simulink model "test_pi_av_flocking_xy_gazebo_2023a"  (R2023a)
settings: Solver=FixedStepAuto  StartTime=0.0  StopTime=inf  FixedStep=0.07  RelTol=1e-3
undefined symbols (not defined in the file or in its folder): angular, DiscIntNeverNeededParam, linear
libraries: ros2lib x14, simulink x4, robotcorelib x4
(part 1 of 2)
settings Model: Creator=johvany  LastModifiedBy=l15
settings OptimizationCC: EnhancedBackFolding=on  PassReuseOutputArgsThreshold=0  ZeroExternalMemoryAtStartup=off  ZeroInternalMemoryAtStartup=off  MaxStackSize=64  OptimizeBlockOrder=speed  DifferentSizesBufferReuse=on  OptimizationCustomize=off
settings DebuggingCC: ParameterTunabilityLossMsg=error  UnderSpecifiedDimensionMsg=warning
settings HardwareCC: ProdBitPerLong=64  ProdHWDeviceType=Intel->x86-64 (Linux 64)  UseEmbeddedCoderFeatures=off
settings SFSimCC: MATLABDynamicMemAlloc=off
settings RTWCC: Description=Embedded Coder  SystemTargetFile=ert.tlc  HardwareBoard=Robot Operating System 2 (ROS 2)  TLCOptions="-aInlineSetEventsForThisBaseRateFcn=TLC_FALSE -aSuppressMultiTaskScheduler=TLC_FALSE  -aRateBasedStepFcn=0"  TemplateMakefile=ert_default_tmf  Toolchain=Colcon Tools  TargetLang=C++
settings CodeAppCC: ForceParamTrailComments=on  OperatorAnnotations=on
settings ERTTargetCC: ERTCustomFileBanners=off  CodeInterfacePackaging=C++ class  SupportContinuousTime=on  SupportNonInlinedSFcns=on  RemoveResetFunc=off  ModelStepFunctionPrototypeControlCompliant=off  RootIOFormat=Structure reference

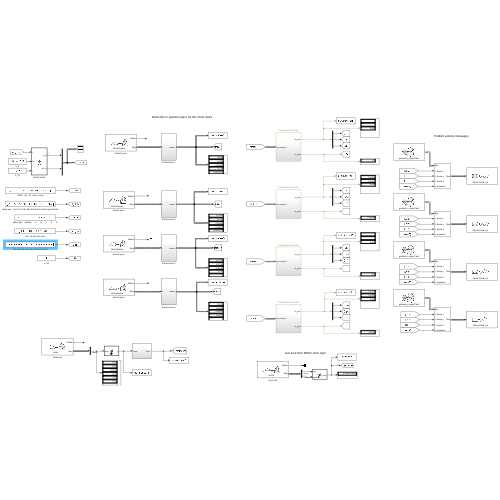
[thumbnail: Simulink's stored preview of the top-level diagram]
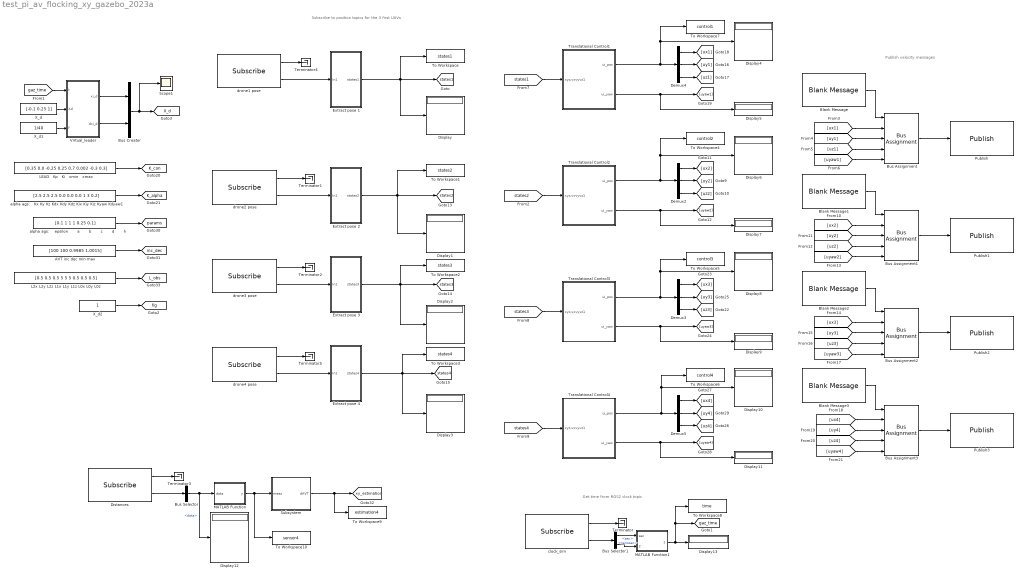
== system test_pi_av_flocking_xy_gazebo_2023a ==
  note: Publish velocity messages
  note: Subscribe to position topics for the 3 first UAVs
  note: Get time from ROS2 clock topic
  AVT inc dec min max : Constant  Value=[100 100 0.9985 1.0015]
  Blank Message{,1..3} (4 alike) : ros2lib/Blank Message  messageClass=Message  entityType=geometry_msgs/Twist  messageType=geometry_msgs/Twist  SampleTime=inf
  Bus Assignment{,1..3} (4 alike) : BusAssignment  AssignedSignals=linear.x,linear.y,linear.z,angular.z
  Bus Creator : BusCreator  Inputs=2
  Bus Selector : BusSelector  OutputSignals=data
  Bus Selector1 : BusSelector  OutputSignals=clock.sec,clock.nanosec
  Demux{2..5} (4 alike) : Demux  Outputs=3
  Display{,1..13} (14 alike) : Display
      Display13 settings: Decimation=4
  Distances : ros2lib/Subscribe  topicSource=Select from ROS network  topic=/dists  messageType=std_msgs/Float32MultiArray  sampleTime=-1  QOSHistory=Keep last  QOSDepth=1  QOSReliability=Reliable  QOSDurability=Volatile
  Extract pose 1 : Subsystem
  Extract pose 2 : Subsystem
  Extract pose 3 : Subsystem
  Extract pose 4 : Subsystem
  L2x L2y L2z L1x L1y L1z L0x L0y L0z : Constant  Value=[0.5 0.5 0.5 5 5 5 0.5 0.5 0.5]
  LEAD   Kp   Ki   xmin   xmax : Constant  Value=[0.35 0.0 -0.25 0.25 0.7 0.002 -0.3 0.3]
  MATLAB Function : MATLAB Function  TreatAsAtomicUnit=on
  MATLAB Function1 : MATLAB Function  TreatAsAtomicUnit=on
  Publish : ros2lib/Publish  topicSource=Select from ROS network  topic=/drone1/cmd_vel  messageType=geometry_msgs/Twist  QOSHistory=Keep last  QOSDepth=1  QOSReliability=Reliable  QOSDurability=Volatile
  Publish1 : ros2lib/Publish  topicSource=Select from ROS network  topic=/drone2/cmd_vel  messageType=geometry_msgs/Twist  QOSHistory=Keep last  QOSDepth=1  QOSReliability=Reliable  QOSDurability=Volatile
  Publish2 : ros2lib/Publish  topicSource=Select from ROS network  topic=/drone3/cmd_vel  messageType=geometry_msgs/Twist  QOSHistory=Keep last  QOSDepth=1  QOSReliability=Reliable  QOSDurability=Volatile
  Publish3 : ros2lib/Publish  topicSource=Select from ROS network  topic=/drone4/cmd_vel  messageType=geometry_msgs/Twist  QOSHistory=Keep last  QOSDepth=1  QOSReliability=Reliable  QOSDurability=Volatile
  Scope1 : Scope
  Subsystem : Subsystem
  Terminator{,1..5} (6 alike) : Terminator
  To Workspace : ToWorkspace  VariableName=states1  SampleTime=-1
  To Workspace1 : ToWorkspace  VariableName=states2  SampleTime=-1
  To Workspace10 : ToWorkspace  VariableName=sensor4  SampleTime=-1
  To Workspace2 : ToWorkspace  VariableName=states3  SampleTime=-1
  To Workspace3 : ToWorkspace  VariableName=states4  SampleTime=-1
  To Workspace4 : ToWorkspace  VariableName=control2  SampleTime=-1
  To Workspace5 : ToWorkspace  VariableName=control3  SampleTime=-1
  To Workspace6 : ToWorkspace  VariableName=control4  SampleTime=-1
  To Workspace7 : ToWorkspace  VariableName=control1  SampleTime=-1
  To Workspace8 : ToWorkspace  VariableName=time  SampleTime=-1
  To Workspace9 : ToWorkspace  VariableName=estimation4  SampleTime=-1
  Translational Control1 : Subsystem
  Translational Control2 : Subsystem
  Translational Control3 : Subsystem
  Translational Control4 : Subsystem
  Virtual_leader : MATLAB Function  TreatAsAtomicUnit=on
  X_d : Constant  Value=[-0.1 0.25 1]
  X_d1 : Constant  Value=1/40
  X_d2 : Constant
  alpha ags:    epsilon       a       b       c       d       h : Constant  Value=[0.1 1 1 1 0.25 0.1]
  alpha ags:   Kx Ky Kz Kdx Kdy Kdz Kix Kiy Kiz Kyaw Kdyaw1 : Constant  Value=[2.5 2.5 2.5 0.0 0.0 0.0 1 3 0.2]
  clock_sim : ros2lib/Subscribe  topicSource=Select from ROS network  topic=/clock  messageType=rosgraph_msgs/Clock  sampleTime=-1  QOSHistory=Keep last  QOSDepth=1  QOSReliability=Reliable  QOSDurability=Volatile
  drone1 pose : ros2lib/Subscribe  topicSource=Select from ROS network  topic=/drone1/pose  messageType=geometry_msgs/PoseStamped  sampleTime=-1  QOSHistory=Keep last  QOSDepth=1  QOSReliability=Reliable  QOSDurability=Volatile
  drone2 pose : ros2lib/Subscribe  topicSource=Select from ROS network  topic=/drone2/pose  messageType=geometry_msgs/PoseStamped  sampleTime=-1  QOSHistory=Keep last  QOSDepth=1  QOSReliability=Reliable  QOSDurability=Volatile
  drone3 pose : ros2lib/Subscribe  topicSource=Select from ROS network  topic=/drone3/pose  messageType=geometry_msgs/PoseStamped  sampleTime=-1  QOSHistory=Keep last  QOSDepth=1  QOSReliability=Reliable  QOSDurability=Volatile
  drone4 pose : ros2lib/Subscribe  topicSource=Select from ROS network  topic=/drone4/pose  messageType=geometry_msgs/PoseStamped  sampleTime=-1  QOSHistory=Keep last  QOSDepth=1  QOSReliability=Reliable  QOSDurability=Volatile
  tag scope: K_alpha=global, K_con=global, L_obs=global, X_d=global, fig=global, gaz_time=global, inc_dec=global, params=global, states1=global, states2=global, states3=global, states4=global, xy_estimation=global
  wires:
  clock_sim/1 -> Terminator/1
  drone2 pose/2 -> Extract pose 2/1(In1)
  drone2 pose/1 -> Terminator1/1
  drone3 pose/2 -> Extract pose 3/1(In1)
  drone3 pose/1 -> Terminator2/1
  Blank Message/1 -> Bus Assignment/1
  Bus Assignment/1 -> Publish/1
  Blank Message1/1 -> Bus Assignment1/1
  Bus Assignment1/1 -> Publish1/1
  Blank Message2/1 -> Bus Assignment2/1
  Bus Assignment2/1 -> Publish2/1
  Blank Message3/1 -> Bus Assignment3/1
  Bus Assignment3/1 -> Publish3/1
  Distances/1 -> Terminator3/1
  Distances/2 -> Bus Selector/1
  Bus Selector/1 -> Display12/1, MATLAB Function/1(data)  "<data>"
  MATLAB Function/1(y) -> To Workspace10/1, Subsystem/1(meas)
  clock_sim/2 -> Bus Selector1/1
  Bus Selector1/1 -> MATLAB Function1/1(sec)  "<sec>"
  Bus Selector1/2 -> MATLAB Function1/2(nanosec)  "<nanosec>"
  Virtual_leader/2(dxi_d) -> Bus Creator/2
  Bus Creator/1 -> Scope1/1, [X_d]
  [gaz_time] -> Virtual_leader/1(t)
  Virtual_leader/1(xi_d) -> Bus Creator/1
  drone1 pose/1 -> Terminator4/1
  drone1 pose/2 -> Extract pose 1/1(In1)
  MATLAB Function1/1(gaz_time) -> To Workspace8/1, [gaz_time], Display13/1
  Extract pose 1/1(states1) -> To Workspace/1, Display/1, [states1]
  [ux1] -> Bus Assignment/2
  [uy1] -> Bus Assignment/3
  [uz1] -> Bus Assignment/4
  [uyaw1] -> Bus Assignment/5
  X_d/1 -> Virtual_leader/2(Xd)
  Extract pose 2/1(states2) -> To Workspace1/1, Display1/1, [states2]
  Extract pose 3/1(states3) -> To Workspace2/1, Display2/1, [states3]
  drone4 pose/2 -> Extract pose 4/1(In1)
  drone4 pose/1 -> Terminator5/1
  Extract pose 4/1(states4) -> To Workspace3/1, Display3/1, [states4]
  [ux2] -> Bus Assignment1/2
  [uy2] -> Bus Assignment1/3
  [uz2] -> Bus Assignment1/4
  [uyaw2] -> Bus Assignment1/5
  [uy3] -> Bus Assignment2/3
  [uyaw3] -> Bus Assignment2/5
  [uz3] -> Bus Assignment2/4
  [ux3] -> Bus Assignment2/2
  [ux4] -> Bus Assignment3/2
  [uy4] -> Bus Assignment3/3
  [uz4] -> Bus Assignment3/4
  [uyaw4] -> Bus Assignment3/5
  Translational Control1/2(ui_yaw) -> Display5/1, [uyaw1]
  Demux4/2 -> [uy1]
  Demux4/3 -> [uz1]
  [states1] -> Translational Control1/1(xyz,vxvyvz1)
  Translational Control1/1(ui_pos) -> Display4/1, To Workspace7/1, Demux4/1
  Demux4/1 -> [ux1]
  LEAD   Kp   Ki   xmin   xmax/1 -> [K_con]
  alpha ags:   Kx Ky Kz Kdx Kdy Kdz Kix Kiy Kiz Kyaw Kdyaw1/1 -> [K_alpha]
  Demux2/1 -> [ux2]
  [states2] -> Translational Control2/1(xyz,vxvyvz1)
  Demux2/3 -> [uz2]
  Demux2/2 -> [uy2]
  Translational Control3/2(ui_yaw) -> Display9/1, [uyaw3]
  Demux3/2 -> [uy3]
  Demux3/3 -> [uz3]
  [states3] -> Translational Control3/1(xyz,vxvyvz1)
  Translational Control3/1(ui_pos) -> To Workspace5/1, Display8/1, Demux3/1
  Demux3/1 -> [ux3]
  Demux5/1 -> [ux4]
  Translational Control4/1(ui_pos) -> To Workspace6/1, Display10/1, Demux5/1
  [states4] -> Translational Control4/1(xyz,vxvyvz1)
  Demux5/3 -> [uz4]
  Demux5/2 -> [uy4]
  Translational Control4/2(ui_yaw) -> Display11/1, [uyaw4]
  alpha ags:    epsilon       a       b       c       d       h/1 -> [params]
  X_d1/1 -> Virtual_leader/3(f)
  AVT inc dec min max/1 -> [inc_dec]
  Subsystem/1(dAVT) -> To Workspace9/1, [xy_estimation]
  L2x L2y L2z L1x L1y L1z L0x L0y L0z/1 -> [L_obs]
  Translational Control2/2(ui_yaw) -> Display7/1, [uyaw2]
  Translational Control2/1(ui_pos) -> To Workspace4/1, Display6/1, Demux2/1
  X_d2/1 -> [fig]

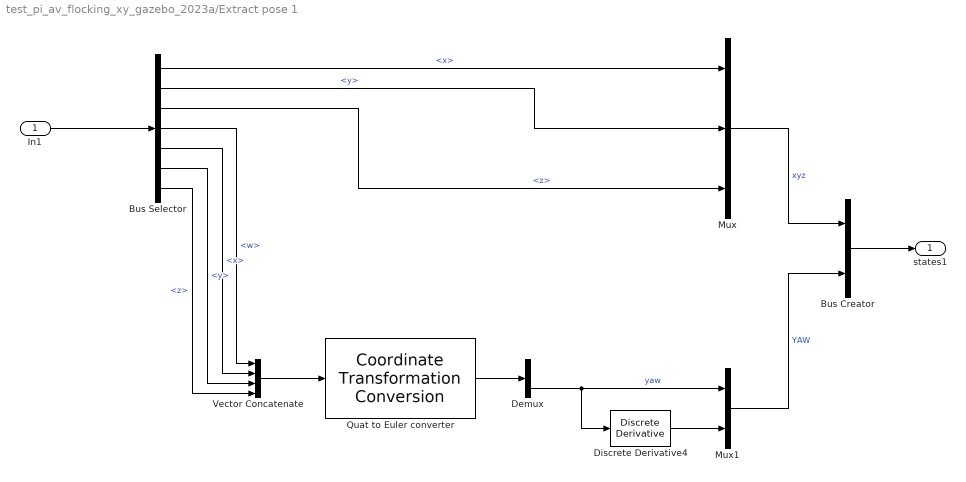
== system test_pi_av_flocking_xy_gazebo_2023a/Extract pose 1 ==
  In1 : Inport
  Bus Creator : BusCreator  Inputs=2
  Bus Selector : BusSelector  OutputSignals=pose.position.x,pose.position.y,pose.position.z,pose.orientation.w,pose.orientation.x,pose.orientation.y,pose.orientation.z
  Demux : Demux  Outputs=3
  Discrete Derivative4 : simulink/Discrete/Discrete Derivative  gainval=1.0  ICPrevScaledInput=0.0  OutMin=[]  OutMax=[]  OutDataType=fixdt(1, 16)  OutScaling=2^-10  DoSatur=off
  Mux : Mux  Inputs=3
  Mux1 : Mux  Inputs=2
  Quat to Euler converter : robotcorelib/Coordinate Transformation Conversion  InputRepresentation=Quaternion  InputEulerSequence=ZYX  ShowTrVecInputPort=on  OutputRepresentation=Euler Angles  OutputEulerSequence=XYZ  ShowTrVecOutputPort=on  SimulateUsing=Interpreted execution
      settings: LibrarySourceBlock=roslib/Utilities/Coordinate Transformation Conversion
  Vector Concatenate : Concatenate  NumInputs=4
  states1 : Outport
  wires:
  Bus Selector/5 -> Vector Concatenate/2  "<x>"
  Quat to Euler converter/1 -> Demux/1
  Bus Selector/6 -> Vector Concatenate/3  "<y>"
  Bus Selector/1 -> Mux/1  "<x>"
  Bus Selector/7 -> Vector Concatenate/4  "<z>"
  Vector Concatenate/1 -> Quat to Euler converter/1
  In1/1 -> Bus Selector/1
  Bus Selector/4 -> Vector Concatenate/1  "<w>"
  Bus Selector/2 -> Mux/2  "<y>"
  Bus Selector/3 -> Mux/3  "<z>"
  Demux/3 -> Discrete Derivative4/1, Mux1/1  "yaw"
  Mux/1 -> Bus Creator/1  "xyz"
  Bus Creator/1 -> states1/1
  Discrete Derivative4/1 -> Mux1/2
  Mux1/1 -> Bus Creator/2  "YAW"

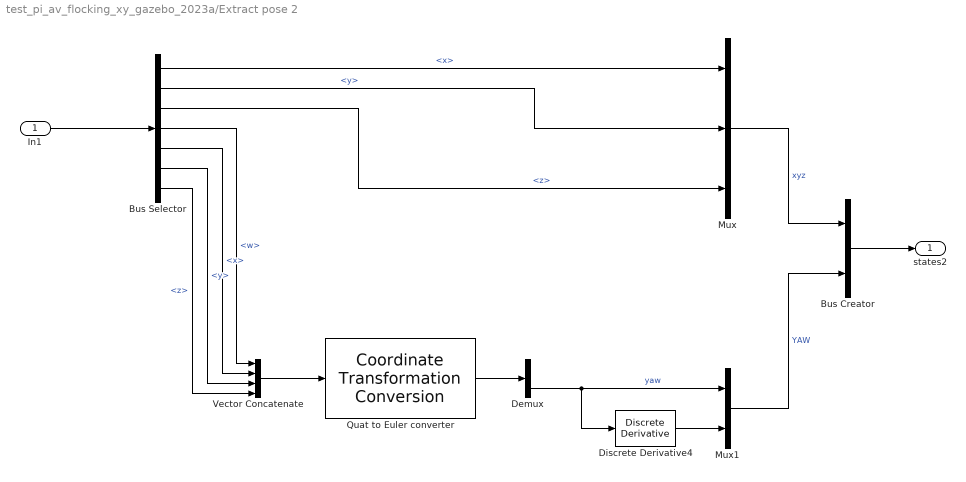
== system test_pi_av_flocking_xy_gazebo_2023a/Extract pose 2 ==
  In1 : Inport
  Bus Creator : BusCreator  Inputs=2
  Bus Selector : BusSelector  OutputSignals=pose.position.x,pose.position.y,pose.position.z,pose.orientation.w,pose.orientation.x,pose.orientation.y,pose.orientation.z
  Demux : Demux  Outputs=3
  Discrete Derivative4 : simulink/Discrete/Discrete Derivative  gainval=1.0  ICPrevScaledInput=0.0  OutMin=[]  OutMax=[]  OutDataType=fixdt(1, 16)  OutScaling=2^-10  DoSatur=off
  Mux : Mux  Inputs=3
  Mux1 : Mux  Inputs=2
  Quat to Euler converter : robotcorelib/Coordinate Transformation Conversion  InputRepresentation=Quaternion  InputEulerSequence=ZYX  ShowTrVecInputPort=on  OutputRepresentation=Euler Angles  OutputEulerSequence=XYZ  ShowTrVecOutputPort=on  SimulateUsing=Interpreted execution
      settings: LibrarySourceBlock=roslib/Utilities/Coordinate Transformation Conversion
  Vector Concatenate : Concatenate  NumInputs=4
  states2 : Outport
  wires:
  Mux1/1 -> Bus Creator/2  "YAW"
  Discrete Derivative4/1 -> Mux1/2
  Bus Creator/1 -> states2/1
  Mux/1 -> Bus Creator/1  "xyz"
  Demux/3 -> Discrete Derivative4/1, Mux1/1  "yaw"
  Bus Selector/3 -> Mux/3  "<z>"
  Bus Selector/2 -> Mux/2  "<y>"
  Bus Selector/4 -> Vector Concatenate/1  "<w>"
  In1/1 -> Bus Selector/1
  Vector Concatenate/1 -> Quat to Euler converter/1
  Bus Selector/7 -> Vector Concatenate/4  "<z>"
  Bus Selector/1 -> Mux/1  "<x>"
  Bus Selector/6 -> Vector Concatenate/3  "<y>"
  Quat to Euler converter/1 -> Demux/1
  Bus Selector/5 -> Vector Concatenate/2  "<x>"

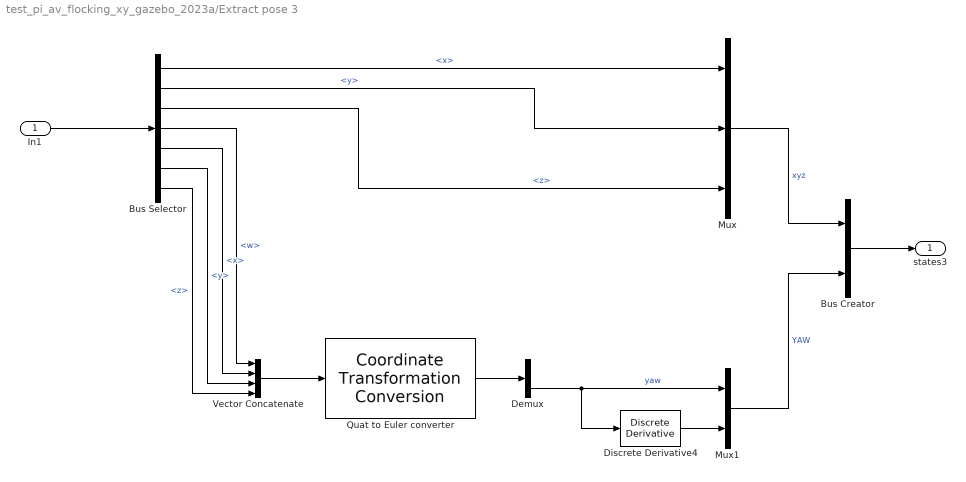
== system test_pi_av_flocking_xy_gazebo_2023a/Extract pose 3 ==
  In1 : Inport
  Bus Creator : BusCreator  Inputs=2
  Bus Selector : BusSelector  OutputSignals=pose.position.x,pose.position.y,pose.position.z,pose.orientation.w,pose.orientation.x,pose.orientation.y,pose.orientation.z
  Demux : Demux  Outputs=3
  Discrete Derivative4 : simulink/Discrete/Discrete Derivative  gainval=1.0  ICPrevScaledInput=0.0  OutMin=[]  OutMax=[]  OutDataType=fixdt(1, 16)  OutScaling=2^-10  DoSatur=off
  Mux : Mux  Inputs=3
  Mux1 : Mux  Inputs=2
  Quat to Euler converter : robotcorelib/Coordinate Transformation Conversion  InputRepresentation=Quaternion  InputEulerSequence=ZYX  ShowTrVecInputPort=on  OutputRepresentation=Euler Angles  OutputEulerSequence=XYZ  ShowTrVecOutputPort=on  SimulateUsing=Interpreted execution
      settings: LibrarySourceBlock=roslib/Utilities/Coordinate Transformation Conversion
  Vector Concatenate : Concatenate  NumInputs=4
  states3 : Outport
  wires:
  Bus Selector/5 -> Vector Concatenate/2  "<x>"
  Quat to Euler converter/1 -> Demux/1
  Bus Selector/6 -> Vector Concatenate/3  "<y>"
  Bus Selector/1 -> Mux/1  "<x>"
  Bus Selector/7 -> Vector Concatenate/4  "<z>"
  Vector Concatenate/1 -> Quat to Euler converter/1
  In1/1 -> Bus Selector/1
  Bus Selector/4 -> Vector Concatenate/1  "<w>"
  Bus Selector/2 -> Mux/2  "<y>"
  Bus Selector/3 -> Mux/3  "<z>"
  Demux/3 -> Discrete Derivative4/1, Mux1/1  "yaw"
  Mux/1 -> Bus Creator/1  "xyz"
  Bus Creator/1 -> states3/1
  Discrete Derivative4/1 -> Mux1/2
  Mux1/1 -> Bus Creator/2  "YAW"

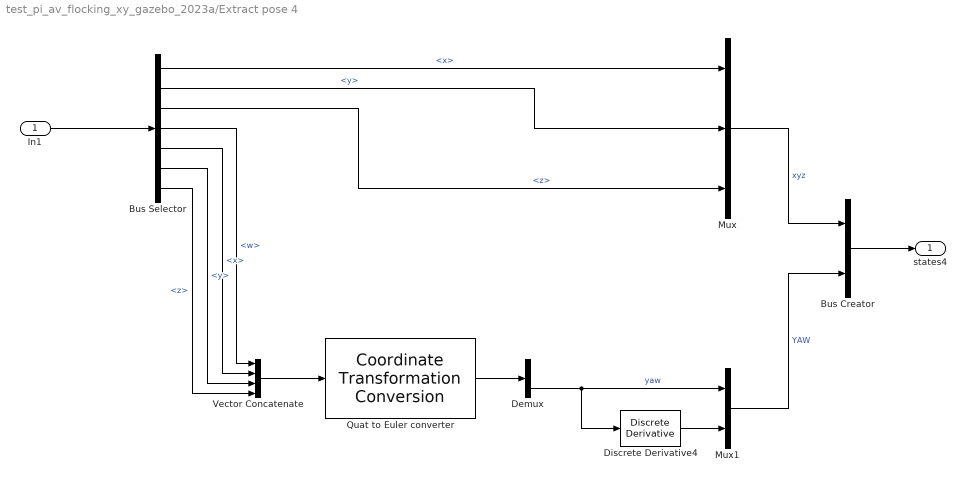
== system test_pi_av_flocking_xy_gazebo_2023a/Extract pose 4 ==
  In1 : Inport
  Bus Creator : BusCreator  Inputs=2
  Bus Selector : BusSelector  OutputSignals=pose.position.x,pose.position.y,pose.position.z,pose.orientation.w,pose.orientation.x,pose.orientation.y,pose.orientation.z
  Demux : Demux  Outputs=3
  Discrete Derivative4 : simulink/Discrete/Discrete Derivative  gainval=1.0  ICPrevScaledInput=0.0  OutMin=[]  OutMax=[]  OutDataType=fixdt(1, 16)  OutScaling=2^-10  DoSatur=off
  Mux : Mux  Inputs=3
  Mux1 : Mux  Inputs=2
  Quat to Euler converter : robotcorelib/Coordinate Transformation Conversion  InputRepresentation=Quaternion  InputEulerSequence=ZYX  ShowTrVecInputPort=on  OutputRepresentation=Euler Angles  OutputEulerSequence=XYZ  ShowTrVecOutputPort=on  SimulateUsing=Interpreted execution
      settings: LibrarySourceBlock=roslib/Utilities/Coordinate Transformation Conversion
  Vector Concatenate : Concatenate  NumInputs=4
  states4 : Outport
  wires:
  Mux1/1 -> Bus Creator/2  "YAW"
  Discrete Derivative4/1 -> Mux1/2
  Bus Creator/1 -> states4/1
  Mux/1 -> Bus Creator/1  "xyz"
  Demux/3 -> Discrete Derivative4/1, Mux1/1  "yaw"
  Bus Selector/3 -> Mux/3  "<z>"
  Bus Selector/2 -> Mux/2  "<y>"
  Bus Selector/4 -> Vector Concatenate/1  "<w>"
  In1/1 -> Bus Selector/1
  Vector Concatenate/1 -> Quat to Euler converter/1
  Bus Selector/7 -> Vector Concatenate/4  "<z>"
  Bus Selector/1 -> Mux/1  "<x>"
  Bus Selector/6 -> Vector Concatenate/3  "<y>"
  Quat to Euler converter/1 -> Demux/1
  Bus Selector/5 -> Vector Concatenate/2  "<x>"

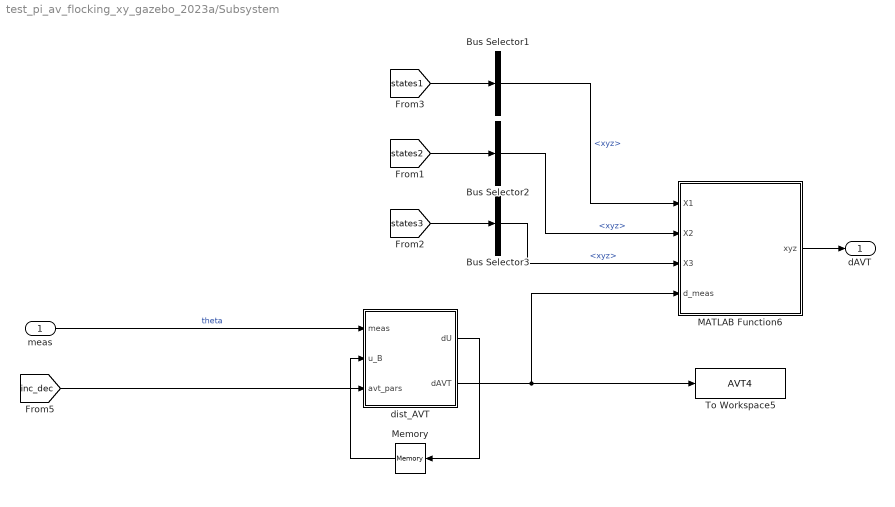
== system test_pi_av_flocking_xy_gazebo_2023a/Subsystem ==
  meas : Inport
  Bus Selector1 : BusSelector  OutputSignals=xyz
  Bus Selector2 : BusSelector  OutputSignals=xyz
  Bus Selector3 : BusSelector  OutputSignals=xyz
  MATLAB Function6 : MATLAB Function  TreatAsAtomicUnit=on
  Memory : Memory  InitialCondition=[1 0.5 0 1 0.5 0 1 0.5 0]
  To Workspace5 : ToWorkspace  VariableName=AVT4  SampleTime=-1
  dist_AVT : MATLAB Function  Tag=Outer control  TreatAsAtomicUnit=on
  dAVT : Outport
  wires:
  Memory/1 -> dist_AVT/2(u_B)
  dist_AVT/2(dAVT) -> To Workspace5/1, MATLAB Function6/4(d_meas)
  dist_AVT/1(dU) -> Memory/1
  meas/1 -> dist_AVT/1(meas)  "theta"
  [inc_dec] -> dist_AVT/3(avt_pars)
  MATLAB Function6/1(xyz) -> dAVT/1
  [states1] -> Bus Selector1/1
  Bus Selector1/1 -> MATLAB Function6/1(X1)  "<xyz>"
  [states2] -> Bus Selector2/1
  [states3] -> Bus Selector3/1
  Bus Selector2/1 -> MATLAB Function6/2(X2)  "<xyz>"
  Bus Selector3/1 -> MATLAB Function6/3(X3)  "<xyz>"

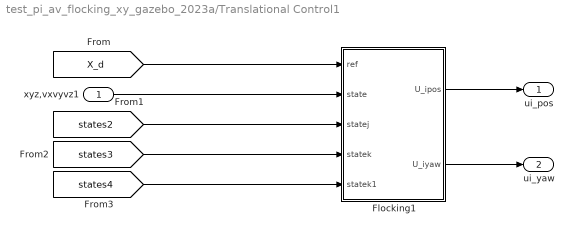
== system test_pi_av_flocking_xy_gazebo_2023a/Translational Control1 ==
  xyz,vxvyvz1 : Inport
  Flocking1 : Subsystem
  ui_pos : Outport  VectorParamsAs1DForOutWhenUnconnected=off
  ui_yaw : Outport  Port=2  VectorParamsAs1DForOutWhenUnconnected=off
  wires:
  [X_d] -> Flocking1/1(ref)
  xyz,vxvyvz1/1 -> Flocking1/2(state)
  [states2] -> Flocking1/3(statej)
  [states3] -> Flocking1/4(statek)
  [states4] -> Flocking1/5(statek1)
  Flocking1/1(U_ipos) -> ui_pos/1
  Flocking1/2(U_iyaw) -> ui_yaw/1

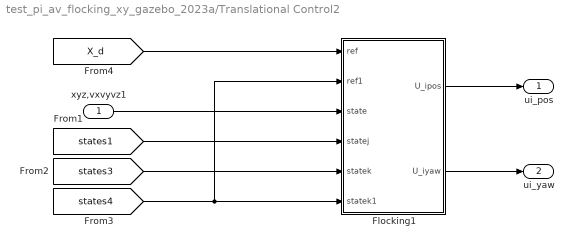
== system test_pi_av_flocking_xy_gazebo_2023a/Translational Control2 ==
  xyz,vxvyvz1 : Inport
  Flocking1 : Subsystem
  ui_pos : Outport  VectorParamsAs1DForOutWhenUnconnected=off
  ui_yaw : Outport  Port=2  VectorParamsAs1DForOutWhenUnconnected=off
  wires:
  Flocking1/2(U_iyaw) -> ui_yaw/1
  Flocking1/1(U_ipos) -> ui_pos/1
  [states4] -> Flocking1/2(ref1), Flocking1/6(statek1)
  [states3] -> Flocking1/5(statek)
  xyz,vxvyvz1/1 -> Flocking1/3(state)
  [states1] -> Flocking1/4(statej)
  [X_d] -> Flocking1/1(ref)

== system test_pi_av_flocking_xy_gazebo_2023a/Translational Control3 ==
  xyz,vxvyvz1 : Inport
  Flocking1 : Subsystem
  ui_pos : Outport  VectorParamsAs1DForOutWhenUnconnected=off
  ui_yaw : Outport  Port=2  VectorParamsAs1DForOutWhenUnconnected=off
  wires:
  [states1] -> Flocking1/4(statej)
  xyz,vxvyvz1/1 -> Flocking1/3(state)
  [states2] -> Flocking1/5(statek)
  [states4] -> Flocking1/2(ref1), Flocking1/6(statek1)
  Flocking1/1(U_ipos) -> ui_pos/1
  Flocking1/2(U_iyaw) -> ui_yaw/1
  [X_d] -> Flocking1/1(ref)

== system test_pi_av_flocking_xy_gazebo_2023a/Translational Control4 ==
  xyz,vxvyvz1 : Inport
  Flocking1 : Subsystem
  ui_pos : Outport  VectorParamsAs1DForOutWhenUnconnected=off
  ui_yaw : Outport  Port=2  VectorParamsAs1DForOutWhenUnconnected=off
  wires:
  Flocking1/2(U_iyaw) -> ui_yaw/1
  Flocking1/1(U_ipos) -> ui_pos/1
  [states3] -> Flocking1/6(statek1)
  [states2] -> Flocking1/5(statek)
  [states1] -> Flocking1/2(ref1), Flocking1/4(statej)
  xyz,vxvyvz1/1 -> Flocking1/3(state)
  [X_d] -> Flocking1/1(ref)

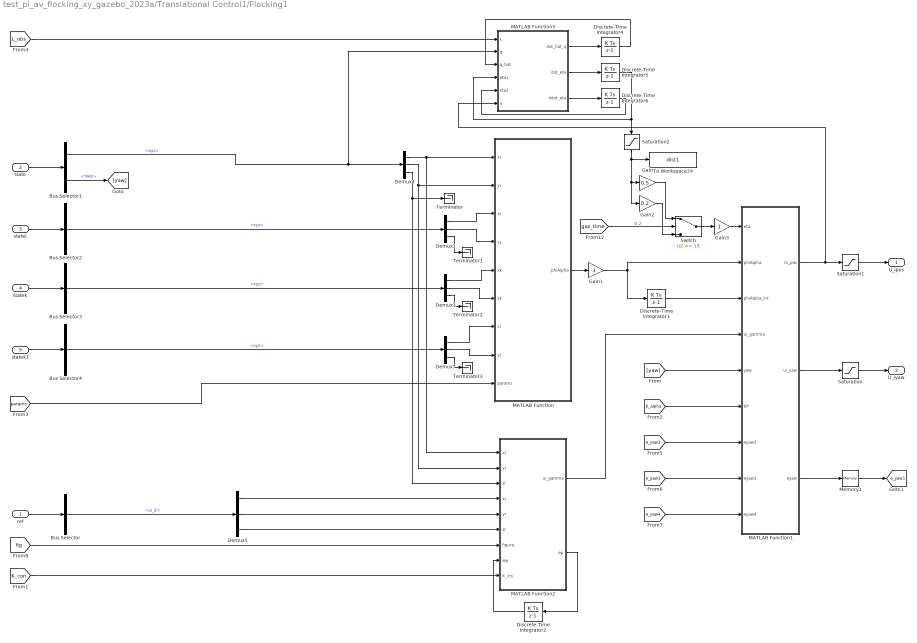
== system test_pi_av_flocking_xy_gazebo_2023a/Translational Control1/Flocking1 ==
  note: 0.2
  ref : Inport
  state : Inport  Port=2
  statej : Inport  Port=3
  statek : Inport  Port=4
  statek1 : Inport  Port=5
  Bus Selector : BusSelector  OutputSignals=xi_d
  Bus Selector1 : BusSelector  OutputSignals=xyz,YAW
  Bus Selector2 : BusSelector  OutputSignals=xyz
  Bus Selector3 : BusSelector  OutputSignals=xyz
  Bus Selector4 : BusSelector  OutputSignals=xyz
  Demux{1,3..5,7} (5 alike) : Demux  Outputs=3
  Discrete-Time Integrator1 : DiscreteIntegrator  SampleTime=-1  LimitOutput=on  UpperSaturationLimit=5  LowerSaturationLimit=-5  ICPrevOutput=DiscIntNeverNeededParam  ICPrevScaledInput=DiscIntNeverNeededParam
  Discrete-Time Integrator2 : DiscreteIntegrator  SampleTime=-1  LimitOutput=on  UpperSaturationLimit=2  LowerSaturationLimit=-2  ICPrevOutput=DiscIntNeverNeededParam  ICPrevScaledInput=DiscIntNeverNeededParam
  Discrete-Time Integrator4 : DiscreteIntegrator  SampleTime=-1  LimitOutput=on  UpperSaturationLimit=0.15  LowerSaturationLimit=-0.15  ICPrevOutput=DiscIntNeverNeededParam  ICPrevScaledInput=DiscIntNeverNeededParam
  Discrete-Time Integrator5 : DiscreteIntegrator  SampleTime=-1  LimitOutput=on  UpperSaturationLimit=0.2  LowerSaturationLimit=-0.2  ICPrevOutput=DiscIntNeverNeededParam  ICPrevScaledInput=DiscIntNeverNeededParam
  Discrete-Time Integrator6 : DiscreteIntegrator  SampleTime=-1  LimitOutput=on  UpperSaturationLimit=0.05  LowerSaturationLimit=-0.05  ICPrevOutput=DiscIntNeverNeededParam  ICPrevScaledInput=DiscIntNeverNeededParam
  Gain : Gain  Gain=0.5
  Gain1 : Gain  Gain=-1
  Gain2 : Gain  Gain=0.2
  Gain3 : Gain
  MATLAB Function : MATLAB Function  TreatAsAtomicUnit=on
  MATLAB Function1 : MATLAB Function  TreatAsAtomicUnit=on
  MATLAB Function2 : MATLAB Function  TreatAsAtomicUnit=on
  MATLAB Function5 : MATLAB Function  TreatAsAtomicUnit=on
  Memory1 : Memory  InitialCondition=1
  Saturation : Saturate  UpperLimit=0.9  LowerLimit=-0.9
  Saturation1 : Saturate  UpperLimit=0.95  LowerLimit=-0.95
  Saturation2 : Saturate  UpperLimit=1  LowerLimit=-1
  Switch : Switch  Threshold=15  SaturateOnIntegerOverflow=off  InputSameDT=off
  Terminator{,1..3} (4 alike) : Terminator
  To Workspace24 : ToWorkspace  VariableName=dist1  SampleTime=-1
  U_ipos : Outport  VectorParamsAs1DForOutWhenUnconnected=off
  U_iyaw : Outport  Port=2  VectorParamsAs1DForOutWhenUnconnected=off
  tag scope: e_yaw1=global
  wires:
  ref/1 -> Bus Selector/1
  state/1 -> Bus Selector1/1
  Bus Selector/1 -> Demux5/1  "<xi_d>"
  statej/1 -> Bus Selector2/1
  Bus Selector2/1 -> Demux1/1  "<xyz>"
  Demux4/1 -> MATLAB Function2/1(xi), MATLAB Function/1(xi)
  Demux4/2 -> MATLAB Function2/2(yi), MATLAB Function/2(yi)
  Demux1/1 -> MATLAB Function/3(xj)
  Demux1/2 -> MATLAB Function/4(yj)
  Discrete-Time Integrator1/1 -> MATLAB Function1/3(phiAlpha_int)
  MATLAB Function2/1(ui_gamma) -> MATLAB Function1/4(ui_gamma)
  statek/1 -> Bus Selector3/1
  Demux3/1 -> MATLAB Function/5(xk)
  Demux3/2 -> MATLAB Function/6(yk)
  Bus Selector3/1 -> Demux3/1  "<xyz>"
  MATLAB Function/1(phiAlpha) -> Gain1/1
  Demux5/1 -> MATLAB Function2/4(xr)
  Demux5/2 -> MATLAB Function2/5(yr)
  Demux4/3 -> Terminator/1, MATLAB Function2/3(zi)
  Demux3/3 -> Terminator2/1
  MATLAB Function1/1(Ui_pos) -> MATLAB Function5/6(u), Saturation1/1
  Demux1/3 -> Terminator1/1
  statek1/1 -> Bus Selector4/1
  Demux7/1 -> MATLAB Function/7(xl)
  Demux7/2 -> MATLAB Function/8(yl)
  Demux7/3 -> Terminator3/1
  Bus Selector4/1 -> Demux7/1  "<xyz>"
  Bus Selector1/1 -> MATLAB Function5/2(q), Demux4/1  "<xyz>"
  Bus Selector1/2 -> [yaw]  "<YAW>"
  [yaw] -> MATLAB Function1/5(yaw)
  MATLAB Function1/2(ui_yaw) -> Saturation/1
  MATLAB Function2/2(ep) -> Discrete-Time Integrator2/1
  Discrete-Time Integrator2/1 -> MATLAB Function2/8(iep)
  [K_con] -> MATLAB Function2/9(K_cts)
  MATLAB Function1/3(eyaw) -> Memory1/1
  [K_alpha] -> MATLAB Function1/6(KP)
  [params] -> MATLAB Function/9(params)
  MATLAB Function5/1(dot_hat_q) -> Discrete-Time Integrator4/1
  Discrete-Time Integrator4/1 -> MATLAB Function5/3(q_hat)
  [L_obs] -> MATLAB Function5/1(L)
  MATLAB Function5/2(dot_eta) -> Discrete-Time Integrator5/1
  MATLAB Function5/3(ddot_eta) -> Discrete-Time Integrator6/1
  Discrete-Time Integrator5/1 -> Saturation2/1, MATLAB Function5/4(eta1)
  Discrete-Time Integrator6/1 -> MATLAB Function5/5(eta2)
  [e_yaw2] -> MATLAB Function1/7(eyaw2)
  [e_yaw3] -> MATLAB Function1/8(eyaw3)
  [e_yaw4] -> MATLAB Function1/9(eyaw4)
  Memory1/1 -> [e_yaw1]
  Saturation/1 -> U_iyaw/1
  Demux5/3 -> MATLAB Function2/6(zr)
  [fig] -> MATLAB Function2/7(figure)
  Gain1/1 -> MATLAB Function1/2(phiAlpha), Discrete-Time Integrator1/1
  Saturation1/1 -> U_ipos/1
  Saturation2/1 -> To Workspace24/1, Gain2/1, Gain/1
  [gaz_time] -> Switch/2
  Gain/1 -> Switch/1
  Gain2/1 -> Switch/3
  Switch/1 -> Gain3/1
  Gain3/1 -> MATLAB Function1/1(eta)

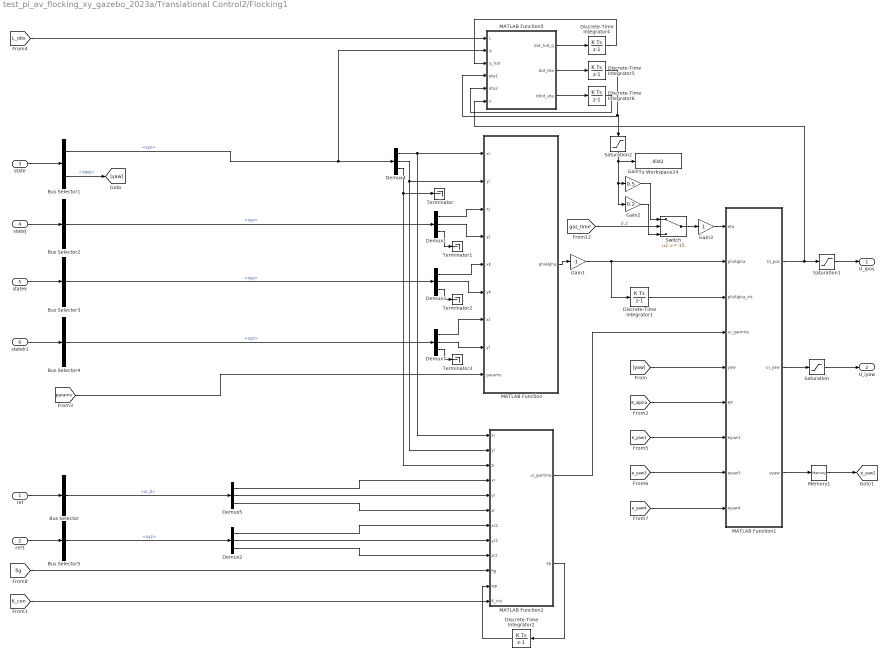
== system test_pi_av_flocking_xy_gazebo_2023a/Translational Control2/Flocking1 ==
  note: 0.2
  ref : Inport
  ref1 : Inport  Port=2
  state : Inport  Port=3
  statej : Inport  Port=4
  statek : Inport  Port=5
  statek1 : Inport  Port=6
  Bus Selector : BusSelector  OutputSignals=xi_d
  Bus Selector1 : BusSelector  OutputSignals=xyz,YAW
  Bus Selector{2..5} (4 alike) : BusSelector  OutputSignals=xyz
  Demux{1..5,7} (6 alike) : Demux  Outputs=3
  Discrete-Time Integrator1 : DiscreteIntegrator  SampleTime=-1  LimitOutput=on  UpperSaturationLimit=5  LowerSaturationLimit=-5  ICPrevOutput=DiscIntNeverNeededParam  ICPrevScaledInput=DiscIntNeverNeededParam
  Discrete-Time Integrator2 : DiscreteIntegrator  SampleTime=-1  LimitOutput=on  UpperSaturationLimit=2  LowerSaturationLimit=-2  ICPrevOutput=DiscIntNeverNeededParam  ICPrevScaledInput=DiscIntNeverNeededParam
  Discrete-Time Integrator4 : DiscreteIntegrator  SampleTime=-1  LimitOutput=on  UpperSaturationLimit=0.15  LowerSaturationLimit=-0.15  ICPrevOutput=DiscIntNeverNeededParam  ICPrevScaledInput=DiscIntNeverNeededParam
  Discrete-Time Integrator5 : DiscreteIntegrator  SampleTime=-1  LimitOutput=on  UpperSaturationLimit=0.2  LowerSaturationLimit=-0.2  ICPrevOutput=DiscIntNeverNeededParam  ICPrevScaledInput=DiscIntNeverNeededParam
  Discrete-Time Integrator6 : DiscreteIntegrator  SampleTime=-1  LimitOutput=on  UpperSaturationLimit=0.05  LowerSaturationLimit=-0.05  ICPrevOutput=DiscIntNeverNeededParam  ICPrevScaledInput=DiscIntNeverNeededParam
  Gain : Gain  Gain=0.5
  Gain1 : Gain  Gain=-1
  Gain2 : Gain  Gain=0.2
  Gain3 : Gain
  MATLAB Function : MATLAB Function  TreatAsAtomicUnit=on
  MATLAB Function1 : MATLAB Function  TreatAsAtomicUnit=on
  MATLAB Function2 : MATLAB Function  TreatAsAtomicUnit=on
  MATLAB Function5 : MATLAB Function  TreatAsAtomicUnit=on
  Memory1 : Memory  InitialCondition=1
  Saturation : Saturate  UpperLimit=0.9  LowerLimit=-0.9
  Saturation1 : Saturate  UpperLimit=0.9  LowerLimit=-0.9
  Saturation2 : Saturate  UpperLimit=1  LowerLimit=-1
  Switch : Switch  Threshold=15  SaturateOnIntegerOverflow=off  InputSameDT=off
  Terminator{,1..3} (4 alike) : Terminator
  To Workspace24 : ToWorkspace  VariableName=dist2  SampleTime=-1
  U_ipos : Outport  VectorParamsAs1DForOutWhenUnconnected=off
  U_iyaw : Outport  Port=2  VectorParamsAs1DForOutWhenUnconnected=off
  tag scope: e_yaw2=global
  wires:
  ref/1 -> Bus Selector/1
  state/1 -> Bus Selector1/1
  Bus Selector/1 -> Demux5/1  "<xi_d>"
  statej/1 -> Bus Selector2/1
  Bus Selector2/1 -> Demux1/1  "<xyz>"
  Demux4/1 -> MATLAB Function2/1(xi), MATLAB Function/1(xi)
  Demux4/2 -> MATLAB Function2/2(yi), MATLAB Function/2(yi)
  Demux1/1 -> MATLAB Function/3(xj)
  Demux1/2 -> MATLAB Function/4(yj)
  Discrete-Time Integrator1/1 -> MATLAB Function1/3(phiAlpha_int)
  MATLAB Function2/1(ui_gamma) -> MATLAB Function1/4(ui_gamma)
  statek/1 -> Bus Selector3/1
  Demux3/1 -> MATLAB Function/5(xk)
  Demux3/2 -> MATLAB Function/6(yk)
  Bus Selector3/1 -> Demux3/1  "<xyz>"
  MATLAB Function/1(phiAlpha) -> Gain1/1
  Demux5/1 -> MATLAB Function2/4(xr)
  Demux5/2 -> MATLAB Function2/5(yr)
  Demux4/3 -> Terminator/1, MATLAB Function2/3(zi)
  Demux3/3 -> Terminator2/1
  MATLAB Function1/1(Ui_pos) -> MATLAB Function5/6(u), Saturation1/1
  Demux1/3 -> Terminator1/1
  statek1/1 -> Bus Selector4/1
  Demux7/1 -> MATLAB Function/7(xl)
  Demux7/2 -> MATLAB Function/8(yl)
  Demux7/3 -> Terminator3/1
  Bus Selector4/1 -> Demux7/1  "<xyz>"
  Bus Selector1/2 -> [yaw]  "<YAW>"
  [yaw] -> MATLAB Function1/5(yaw)
  MATLAB Function1/2(ui_yaw) -> Saturation/1
  MATLAB Function2/2(ep) -> Discrete-Time Integrator2/1
  Discrete-Time Integrator2/1 -> MATLAB Function2/11(iep)
  [K_con] -> MATLAB Function2/12(K_cts)
  MATLAB Function1/3(eyaw) -> Memory1/1
  [K_alpha] -> MATLAB Function1/6(KP)
  [params] -> MATLAB Function/9(params)
  [L_obs] -> MATLAB Function5/1(L)
  MATLAB Function5/1(dot_hat_q) -> Discrete-Time Integrator4/1
  Discrete-Time Integrator4/1 -> MATLAB Function5/3(q_hat)
  MATLAB Function5/2(dot_eta) -> Discrete-Time Integrator5/1
  MATLAB Function5/3(ddot_eta) -> Discrete-Time Integrator6/1
  Discrete-Time Integrator6/1 -> MATLAB Function5/5(eta2)
  Bus Selector1/1 -> MATLAB Function5/2(q), Demux4/1  "<xyz>"
  Discrete-Time Integrator5/1 -> Saturation2/1, MATLAB Function5/4(eta1)
  [e_yaw1] -> MATLAB Function1/7(eyaw1)
  [e_yaw3] -> MATLAB Function1/8(eyaw3)
  [e_yaw4] -> MATLAB Function1/9(eyaw4)
  Memory1/1 -> [e_yaw2]
  Saturation/1 -> U_iyaw/1
  Demux5/3 -> MATLAB Function2/6(zr)
  Bus Selector5/1 -> Demux2/1  "<xyz>"
  ref1/1 -> Bus Selector5/1
  Demux2/1 -> MATLAB Function2/7(xr2)
  Demux2/2 -> MATLAB Function2/8(yr2)
  Demux2/3 -> MATLAB Function2/9(zr2)
  [fig] -> MATLAB Function2/10(fig)
  Gain1/1 -> MATLAB Function1/2(phiAlpha), Discrete-Time Integrator1/1
  Saturation1/1 -> U_ipos/1
  Saturation2/1 -> To Workspace24/1, Gain2/1, Gain/1
  Gain2/1 -> Switch/3
  [gaz_time] -> Switch/2
  Gain/1 -> Switch/1
  Switch/1 -> Gain3/1
  Gain3/1 -> MATLAB Function1/1(eta)

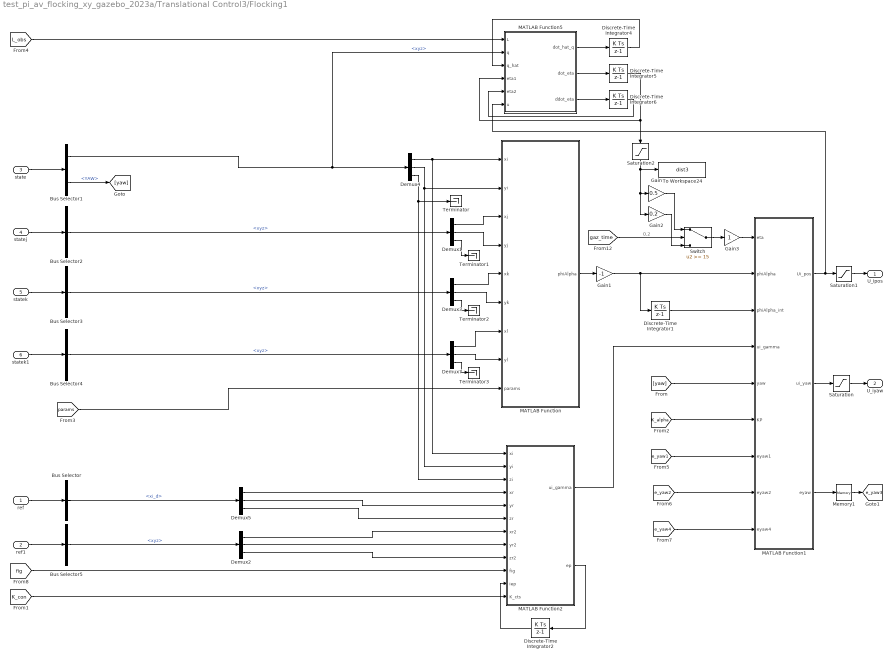
== system test_pi_av_flocking_xy_gazebo_2023a/Translational Control3/Flocking1 ==
  note: 0.2
  ref : Inport
  ref1 : Inport  Port=2
  state : Inport  Port=3
  statej : Inport  Port=4
  statek : Inport  Port=5
  statek1 : Inport  Port=6
  Bus Selector : BusSelector  OutputSignals=xi_d
  Bus Selector1 : BusSelector  OutputSignals=xyz,YAW
  Bus Selector{2..5} (4 alike) : BusSelector  OutputSignals=xyz
  Demux{1..5,7} (6 alike) : Demux  Outputs=3
  Discrete-Time Integrator1 : DiscreteIntegrator  SampleTime=-1  LimitOutput=on  UpperSaturationLimit=5  LowerSaturationLimit=-5  ICPrevOutput=DiscIntNeverNeededParam  ICPrevScaledInput=DiscIntNeverNeededParam
  Discrete-Time Integrator2 : DiscreteIntegrator  SampleTime=-1  LimitOutput=on  UpperSaturationLimit=2  LowerSaturationLimit=-2  ICPrevOutput=DiscIntNeverNeededParam  ICPrevScaledInput=DiscIntNeverNeededParam
  Discrete-Time Integrator4 : DiscreteIntegrator  SampleTime=-1  LimitOutput=on  UpperSaturationLimit=0.15  LowerSaturationLimit=-0.15  ICPrevOutput=DiscIntNeverNeededParam  ICPrevScaledInput=DiscIntNeverNeededParam
  Discrete-Time Integrator5 : DiscreteIntegrator  SampleTime=-1  LimitOutput=on  UpperSaturationLimit=0.2  LowerSaturationLimit=-0.2  ICPrevOutput=DiscIntNeverNeededParam  ICPrevScaledInput=DiscIntNeverNeededParam
  Discrete-Time Integrator6 : DiscreteIntegrator  SampleTime=-1  LimitOutput=on  UpperSaturationLimit=0.05  LowerSaturationLimit=-0.05  ICPrevOutput=DiscIntNeverNeededParam  ICPrevScaledInput=DiscIntNeverNeededParam
  Gain : Gain  Gain=0.5
  Gain1 : Gain  Gain=-1
  Gain2 : Gain  Gain=0.2
  Gain3 : Gain
  MATLAB Function : MATLAB Function  TreatAsAtomicUnit=on
  MATLAB Function1 : MATLAB Function  TreatAsAtomicUnit=on
  MATLAB Function2 : MATLAB Function  TreatAsAtomicUnit=on
  MATLAB Function5 : MATLAB Function  TreatAsAtomicUnit=on
  Memory1 : Memory  InitialCondition=1
  Saturation : Saturate  UpperLimit=0.9  LowerLimit=-0.9
  Saturation1 : Saturate  UpperLimit=0.9  LowerLimit=-0.9
  Saturation2 : Saturate  UpperLimit=1  LowerLimit=-1
  Switch : Switch  Threshold=15  SaturateOnIntegerOverflow=off  InputSameDT=off
  Terminator{,1..3} (4 alike) : Terminator
  To Workspace24 : ToWorkspace  VariableName=dist3  SampleTime=-1
  U_ipos : Outport  VectorParamsAs1DForOutWhenUnconnected=off
  U_iyaw : Outport  Port=2  VectorParamsAs1DForOutWhenUnconnected=off
  tag scope: e_yaw3=global
  wires:
  ref/1 -> Bus Selector/1
  state/1 -> Bus Selector1/1
  Bus Selector/1 -> Demux5/1  "<xi_d>"
  statej/1 -> Bus Selector2/1
  Bus Selector2/1 -> Demux1/1  "<xyz>"
  Demux4/1 -> MATLAB Function2/1(xi), MATLAB Function/1(xi)
  Demux4/2 -> MATLAB Function2/2(yi), MATLAB Function/2(yi)
  Demux1/1 -> MATLAB Function/3(xj)
  Demux1/2 -> MATLAB Function/4(yj)
  Discrete-Time Integrator1/1 -> MATLAB Function1/3(phiAlpha_int)
  MATLAB Function2/1(ui_gamma) -> MATLAB Function1/4(ui_gamma)
  statek/1 -> Bus Selector3/1
  Demux3/1 -> MATLAB Function/5(xk)
  Demux3/2 -> MATLAB Function/6(yk)
  Bus Selector3/1 -> Demux3/1  "<xyz>"
  MATLAB Function/1(phiAlpha) -> Gain1/1
  Demux5/1 -> MATLAB Function2/4(xr)
  Demux5/2 -> MATLAB Function2/5(yr)
  Demux4/3 -> Terminator/1, MATLAB Function2/3(zi)
  Demux3/3 -> Terminator2/1
  MATLAB Function1/1(Ui_pos) -> MATLAB Function5/6(u), Saturation1/1
  Demux1/3 -> Terminator1/1
  statek1/1 -> Bus Selector4/1
  Demux7/1 -> MATLAB Function/7(xl)
  Demux7/2 -> MATLAB Function/8(yl)
  Demux7/3 -> Terminator3/1
  Bus Selector4/1 -> Demux7/1  "<xyz>"
  Bus Selector1/1 -> MATLAB Function5/2(q), Demux4/1  "<xyz>"
  Bus Selector1/2 -> [yaw]  "<YAW>"
  [yaw] -> MATLAB Function1/5(yaw)
  MATLAB Function1/2(ui_yaw) -> Saturation/1
  MATLAB Function2/2(ep) -> Discrete-Time Integrator2/1
  Discrete-Time Integrator2/1 -> MATLAB Function2/11(iep)
  [K_con] -> MATLAB Function2/12(K_cts)
  MATLAB Function1/3(eyaw) -> Memory1/1
  [K_alpha] -> MATLAB Function1/6(KP)
  [params] -> MATLAB Function/9(params)
  Discrete-Time Integrator6/1 -> MATLAB Function5/5(eta2)
  MATLAB Function5/3(ddot_eta) -> Discrete-Time Integrator6/1
  Discrete-Time Integrator4/1 -> MATLAB Function5/3(q_hat)
  MATLAB Function5/2(dot_eta) -> Discrete-Time Integrator5/1
  MATLAB Function5/1(dot_hat_q) -> Discrete-Time Integrator4/1
  [L_obs] -> MATLAB Function5/1(L)
  Discrete-Time Integrator5/1 -> Saturation2/1, MATLAB Function5/4(eta1)
  [e_yaw2] -> MATLAB Function1/8(eyaw2)
  [e_yaw4] -> MATLAB Function1/9(eyaw4)
  [e_yaw1] -> MATLAB Function1/7(eyaw1)
  Memory1/1 -> [e_yaw3]
  Saturation/1 -> U_iyaw/1
  Demux5/3 -> MATLAB Function2/6(zr)
  Bus Selector5/1 -> Demux2/1  "<xyz>"
  ref1/1 -> Bus Selector5/1
  Demux2/3 -> MATLAB Function2/9(zr2)
  Demux2/2 -> MATLAB Function2/8(yr2)
  Demux2/1 -> MATLAB Function2/7(xr2)
  [fig] -> MATLAB Function2/10(fig)
  Gain1/1 -> MATLAB Function1/2(phiAlpha), Discrete-Time Integrator1/1
  Saturation1/1 -> U_ipos/1
  Saturation2/1 -> To Workspace24/1, Gain2/1, Gain/1
  Gain2/1 -> Switch/3
  [gaz_time] -> Switch/2
  Gain/1 -> Switch/1
  Switch/1 -> Gain3/1
  Gain3/1 -> MATLAB Function1/1(eta)

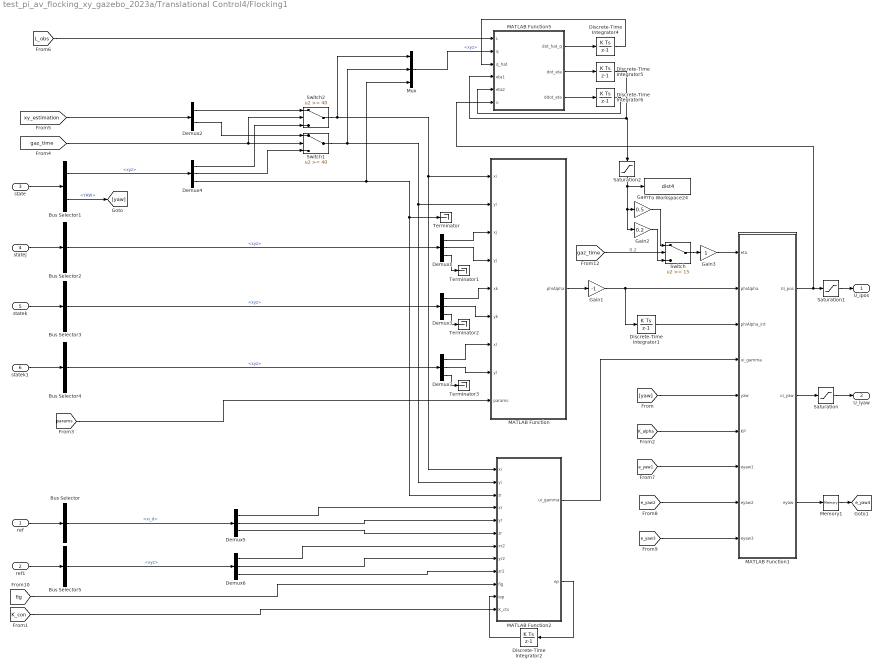
== system test_pi_av_flocking_xy_gazebo_2023a/Translational Control4/Flocking1 ==
  note: 0.2
  ref : Inport
  ref1 : Inport  Port=2
  state : Inport  Port=3
  statej : Inport  Port=4
  statek : Inport  Port=5
  statek1 : Inport  Port=6
  Bus Selector : BusSelector  OutputSignals=xi_d
  Bus Selector1 : BusSelector  OutputSignals=xyz,YAW
  Bus Selector{2..5} (4 alike) : BusSelector  OutputSignals=xyz
  Demux{1,3..7} (6 alike) : Demux  Outputs=3
  Demux2 : Demux  Outputs=2
  Discrete-Time Integrator1 : DiscreteIntegrator  SampleTime=-1  LimitOutput=on  UpperSaturationLimit=5  LowerSaturationLimit=-5  ICPrevOutput=DiscIntNeverNeededParam  ICPrevScaledInput=DiscIntNeverNeededParam
  Discrete-Time Integrator2 : DiscreteIntegrator  SampleTime=-1  LimitOutput=on  UpperSaturationLimit=2  LowerSaturationLimit=-2  ICPrevOutput=DiscIntNeverNeededParam  ICPrevScaledInput=DiscIntNeverNeededParam
  Discrete-Time Integrator4 : DiscreteIntegrator  SampleTime=-1  LimitOutput=on  UpperSaturationLimit=0.15  LowerSaturationLimit=-0.15  ICPrevOutput=DiscIntNeverNeededParam  ICPrevScaledInput=DiscIntNeverNeededParam
  Discrete-Time Integrator5 : DiscreteIntegrator  SampleTime=-1  LimitOutput=on  UpperSaturationLimit=0.2  LowerSaturationLimit=-0.2  ICPrevOutput=DiscIntNeverNeededParam  ICPrevScaledInput=DiscIntNeverNeededParam
  Discrete-Time Integrator6 : DiscreteIntegrator  SampleTime=-1  LimitOutput=on  UpperSaturationLimit=0.05  LowerSaturationLimit=-0.05  ICPrevOutput=DiscIntNeverNeededParam  ICPrevScaledInput=DiscIntNeverNeededParam
  Gain : Gain  Gain=0.5
  Gain1 : Gain  Gain=-1
  Gain2 : Gain  Gain=0.2
  Gain3 : Gain
  MATLAB Function : MATLAB Function  TreatAsAtomicUnit=on
  MATLAB Function1 : MATLAB Function  TreatAsAtomicUnit=on
  MATLAB Function2 : MATLAB Function  TreatAsAtomicUnit=on
  MATLAB Function5 : MATLAB Function  TreatAsAtomicUnit=on
  Memory1 : Memory  InitialCondition=1
  Mux : Mux  Inputs=3
  Saturation : Saturate  UpperLimit=0.9  LowerLimit=-0.9
  Saturation1 : Saturate  UpperLimit=0.9  LowerLimit=-0.9
  Saturation2 : Saturate  UpperLimit=1  LowerLimit=-1
  Switch : Switch  Threshold=15  SaturateOnIntegerOverflow=off  InputSameDT=off
  Switch1 : Switch  Threshold=40  SaturateOnIntegerOverflow=off  InputSameDT=off
  Switch2 : Switch  Threshold=40  SaturateOnIntegerOverflow=off  InputSameDT=off
  Terminator{,1..3} (4 alike) : Terminator
  To Workspace24 : ToWorkspace  VariableName=dist4  SampleTime=-1
  U_ipos : Outport  VectorParamsAs1DForOutWhenUnconnected=off
  U_iyaw : Outport  Port=2  VectorParamsAs1DForOutWhenUnconnected=off
  tag scope: e_yaw4=global
  wires:
  ref/1 -> Bus Selector/1
  state/1 -> Bus Selector1/1
  Bus Selector/1 -> Demux5/1  "<xi_d>"
  statej/1 -> Bus Selector2/1
  Bus Selector2/1 -> Demux1/1  "<xyz>"
  Demux1/1 -> MATLAB Function/3(xj)
  Demux1/2 -> MATLAB Function/4(yj)
  Discrete-Time Integrator1/1 -> MATLAB Function1/3(phiAlpha_int)
  MATLAB Function2/1(ui_gamma) -> MATLAB Function1/4(ui_gamma)
  statek/1 -> Bus Selector3/1
  Demux3/1 -> MATLAB Function/5(xk)
  Demux3/2 -> MATLAB Function/6(yk)
  Bus Selector3/1 -> Demux3/1  "<xyz>"
  MATLAB Function/1(phiAlpha) -> Gain1/1
  Demux5/1 -> MATLAB Function2/4(xr)
  Demux5/2 -> MATLAB Function2/5(yr)
  Demux4/3 -> Mux/3, Terminator/1, MATLAB Function2/3(zi)
  Demux3/3 -> Terminator2/1
  MATLAB Function1/1(Ui_pos) -> MATLAB Function5/6(u), Saturation1/1
  Demux1/3 -> Terminator1/1
  statek1/1 -> Bus Selector4/1
  Demux7/1 -> MATLAB Function/7(xl)
  Demux7/2 -> MATLAB Function/8(yl)
  Demux7/3 -> Terminator3/1
  Bus Selector4/1 -> Demux7/1  "<xyz>"
  Bus Selector1/2 -> [yaw]  "<YAW>"
  [yaw] -> MATLAB Function1/5(yaw)
  MATLAB Function1/2(ui_yaw) -> Saturation/1
  MATLAB Function2/2(ep) -> Discrete-Time Integrator2/1
  Discrete-Time Integrator2/1 -> MATLAB Function2/11(iep)
  [K_con] -> MATLAB Function2/12(K_cts)
  MATLAB Function1/3(eyaw) -> Memory1/1
  [K_alpha] -> MATLAB Function1/6(KP)
  [params] -> MATLAB Function/9(params)
  Bus Selector1/1 -> Demux4/1  "<xyz>"
  [xy_estimation] -> Demux2/1
  [gaz_time] -> Switch1/2, Switch2/2
  Switch2/1 -> MATLAB Function2/1(xi), MATLAB Function/1(xi), Mux/1
  Switch1/1 -> MATLAB Function/2(yi), MATLAB Function2/2(yi), Mux/2
  Demux2/1 -> Switch2/1
  Demux2/2 -> Switch1/1
  [L_obs] -> MATLAB Function5/1(L)
  Discrete-Time Integrator4/1 -> MATLAB Function5/3(q_hat)
  MATLAB Function5/2(dot_eta) -> Discrete-Time Integrator5/1
  Discrete-Time Integrator5/1 -> Saturation2/1, MATLAB Function5/4(eta1)
  MATLAB Function5/3(ddot_eta) -> Discrete-Time Integrator6/1
  Discrete-Time Integrator6/1 -> MATLAB Function5/5(eta2)
  MATLAB Function5/1(dot_hat_q) -> Discrete-Time Integrator4/1
  Mux/1 -> MATLAB Function5/2(q)  "<xyz>"
  [e_yaw1] -> MATLAB Function1/7(eyaw1)
  [e_yaw2] -> MATLAB Function1/8(eyaw2)
  [e_yaw3] -> MATLAB Function1/9(eyaw3)
  Memory1/1 -> [e_yaw4]
  Demux4/1 -> Switch2/3
  Demux4/2 -> Switch1/3
  Saturation/1 -> U_iyaw/1
  Demux5/3 -> MATLAB Function2/6(zr)
  Bus Selector5/1 -> Demux6/1  "<xyz>"
  ref1/1 -> Bus Selector5/1
  Demux6/2 -> MATLAB Function2/8(yr2)
  Demux6/1 -> MATLAB Function2/7(xr2)
  Demux6/3 -> MATLAB Function2/9(zr2)
  Gain1/1 -> MATLAB Function1/2(phiAlpha), Discrete-Time Integrator1/1
  Saturation1/1 -> U_ipos/1
  [fig] -> MATLAB Function2/10(fig)
  Saturation2/1 -> To Workspace24/1, Gain2/1, Gain/1
  Gain2/1 -> Switch/3
  [gaz_time] -> Switch/2
  Gain/1 -> Switch/1
  Switch/1 -> Gain3/1
  Gain3/1 -> MATLAB Function1/1(eta)

== matlab function test_pi_av_flocking_xy_gazebo_2023a/MATLAB Function ==
  data: data input; y output
function y = fcn(data)

%DATA = data(1:20);
d1 = double(data(4));
d2 = double(data(5));
d3 = double(data(6));
y = [d1;d2;d3];

== matlab function test_pi_av_flocking_xy_gazebo_2023a/Virtual_leader ==
  data: t input; xi_d output; dxi_d output; Xd input; f input
function [xi_d, dxi_d]  = fcn(t, Xd, f)
%#codegen



%f=1/60;    %freq in Hz
radius=1;   %radius in meters

sel=2;      %inputs or parameters dont work! only local vars ...

if sel == 1
    if t < 90
       xd     =  0.4;
       xdotd  =  0;
           
       yd     = 0.4;
       ydotd  = 0;
           
       zd     = 0.7;  
       zdotd  = 0; 
           
       xi_d =[xd; yd; zd];
       dxi_d=[xdotd; ydotd; zdotd]; 
       
    elseif t < 120
        xd     =  0.4;
        xdotd  =  0;
            
        yd     = -0.4;
        ydotd  = 0;
            
        zd     = 0.7;  
        zdotd  = 0; 
            
        xi_d =[xd; yd; zd];
        dxi_d=[xdotd; ydotd; zdotd]; 
        
    else
       xd     = radius*sin(2*pi*f*t);
       xdotd  = radius*2*pi*f*cos(2*pi*f*t);
            
       yd     = radius*cos(2*pi*f*t);
       ydotd  = -radius*2*pi*f*sin(2*pi*f*t);
            
       zd     = 0.7;  %radius*cos(2*pi*f*t) + 5;
       zdotd  = 0;  %-radius*2*pi*f*sin(2*pi*f*t);
           
       xi_d =[xd; yd; zd];
       dxi_d=[xdotd; ydotd; zdotd];
       
    end
end

 if(sel==2)
     xd     =  Xd(1);
     xdotd  =  0;
          
     yd     = Xd(2);
     ydotd  = 0;
          
     zd     = Xd(3);  
     zdotd  = 0; 
          
     xi_d =[xd; yd; zd];
     dxi_d=[xdotd; ydotd; zdotd]; 
     
 end

== matlab function test_pi_av_flocking_xy_gazebo_2023a/Translational Control2/Flocking1/MATLAB Function ==
  data: xi input; yi input; phiAlpha output; xj input; yj input; xk input; yk input; xl input; yl input; params input

function phiAlpha  = phiAlphaFcn(xi, yi, xj, yj, xk, yk, xl, yl, params)
    
    % Flocking parameters
    epsilon = params(1); a = params(2); b = params(3); c = params(4); d = params(5); h = params(6);

    e = abs(a - b) / sqrt(4*a*b) ;

    cAlpha = sigmaNormFun(c, epsilon) ;
    dAlpha = sigmaNormFun(d, epsilon) ;

    %%
    Pi = [xi;yi] ;
    Pj = [xj;yj] ;
    Pk = [xk;yk] ;
    Pl = [xl;yl] ;

    %%
    sigmaNormj = sigmaNormFun(Pj - Pi, epsilon) ;
    nij = gradSigmaFun(Pj - Pi, epsilon) ;
    
    sigmaNormk = sigmaNormFun(Pk - Pi, epsilon) ;
    nik = gradSigmaFun(Pk - Pi, epsilon) ;

    sigmaNorml = sigmaNormFun(Pl - Pi, epsilon) ;
    nil = gradSigmaFun(Pl - Pi, epsilon) ;

    %%
    sigma1j = sigma1Fun(sigmaNormj - dAlpha + e) ;
    sigma1k = sigma1Fun(sigmaNormk - dAlpha + e) ;
    sigma1l = sigma1Fun(sigmaNorml - dAlpha + e) ;
            
    %% Position
    phiAlphaj = 0.5 * bumpFcn(sigmaNormj/cAlpha,h) * ((a+b)*sigma1j + (a-b)) ;
    phiAlphanij = phiAlphaj.* nij ;
    
    phiAlphak = 0.5 * bumpFcn(sigmaNormk/cAlpha,h) * ((a+b)*sigma1k + (a-b)) ;
    phiAlphanik = phiAlphak.* nik ;

    phiAlphal = 0.5 * bumpFcn(sigmaNorml/cAlpha,h) * ((a+b)*sigma1l + (a-b)) ;
    phiAlphanil = phiAlphal.* nil ;

    phiAlpha = phiAlphanij + phiAlphanik + phiAlphanil;

    
end

== matlab function test_pi_av_flocking_xy_gazebo_2023a/Translational Control2/Flocking1/MATLAB Function1 ==
  data: eta input; phiAlpha input; phiAlpha_int input; ui_gamma input; yaw input; Ui_pos output size=3; ui_yaw output; KP input; eyaw output size=1; eyaw1 input; eyaw3 input; eyaw4 input

function [Ui_pos, ui_yaw, eyaw]  = ctrlLaw(eta, phiAlpha, phiAlpha_int, ui_gamma, yaw, KP, eyaw1, eyaw3, eyaw4)  %, phiBetak, bikobs, phiBetanei, bikve
    
    % Control gains and parameters
    Kx = KP(1); Ky = KP(2); Kz = KP(3);
    Kix = KP(4); Kiy = KP(5); Kiz = KP(6);
    Kyaw = KP(7); Kdyaw = KP(8); 
    off = KP(9);

    eyaw = 0 - yaw(1);
    deyaw = 0 - yaw(2);


    ui_yaw = Kyaw*eyaw + Kdyaw*deyaw;
    hz_dot = ui_gamma(3,1) - eta(3,1);  %+ cBetaz * (phiBetak(3,1) + phiBetanei(3,1)) + cdBetaz * (bikobs(3,1) + bikve(3,1));

    if eyaw < off && eyaw > -off % && eyaw1 < off && eyaw1 > -off && eyaw3 < off && eyaw3 > -off && eyaw4 < off && eyaw4 > -off
        hx_dot = Kx * phiAlpha(1,1) + Kix * phiAlpha_int(1,1) + ui_gamma(1,1) - eta(1,1);  %+ cBetax * (phiBetak(1,1) + phiBetanei(1,1)) + cdBetax * (bikobs(1,1) + bikve(1,1));
        hy_dot = Ky * phiAlpha(2,1) + Kiy * phiAlpha_int(2,1) + ui_gamma(2,1) - eta(2,1);  %+ cBetay * (phiBetak(2,1) + phiBetanei(2,1)) + cdBetay * (bikobs(2,1) + bikve(2,1));
    else
        hx_dot = 0;
        hy_dot = 0;
    end
    

    Ui_pos = [hx_dot; hy_dot; hz_dot] ;
    

end

== matlab function test_pi_av_flocking_xy_gazebo_2023a/Translational Control2/Flocking1/MATLAB Function2 ==
  data: xi input; yi input; zi input; ui_gamma output; xr input; yr input; zr input; xr2 input; yr2 input; zr2 input; fig input; iep input size=3; ep output size=3; K_cts input

function [ui_gamma, ep] = naviFeedback(xi, yi, zi, xr, yr, zr, xr2, yr2, zr2, fig, iep, K_cts)
    
    Kpxy = K_cts(1); Kixy = K_cts(2);
    xminxy = K_cts(3); xmaxxy = K_cts(4);
    Kpz = K_cts(5); Kiz = K_cts(6);
    xminz = K_cts(7); xmaxz = K_cts(8);
    
    if fig == 1
        e_x = (xr - xi - 0.5) + (xr2 - xi - 1);
        e_y = (yr - yi + 0.5) + (yr2 - yi + 1);
        e_z = (zr - zi - 0.1) + (zr2 - zi);
    elseif fig == 2
        e_x = (xr - xi - 0.5) + (xr2 - xi - 1);
        e_y = (yr - yi - 0.5) + (yr2 - yi - 1);
        e_z = (zr - zi + 0.1) + (zr2 - zi);
    else
        e_x = (xr - xi - 0.5) + (xr2 - xi - 1);
        e_y = (yr - yi - 0.5) + (yr2 - yi - 1);
        e_z = (zr - zi + 0.1) + (zr2 - zi);
    end

    e_xy = [e_x;e_y];
    ep = [e_xy;e_z];
    
    ui_xy = satFcn_xy(Kpxy.*(e_xy), xminxy, xmaxxy) + satFcn_xy(Kixy.*([iep(1);iep(2)]), xminxy, xmaxxy) ;
    ui_z = satFcn_z(Kpz*(e_z), xminz, xmaxz) + satFcn_z(Kiz*(iep(3)), xminz, xmaxz) ;

    ui_gamma = [ui_xy;ui_z];    
    
end

== matlab function test_pi_av_flocking_xy_gazebo_2023a/Translational Control3/Flocking1/MATLAB Function ==
  data: xi input; yi input; phiAlpha output; xj input; yj input; xk input; yk input; xl input; yl input; params input

function phiAlpha  = phiAlphaFcn(xi, yi, xj, yj, xk, yk, xl, yl, params)
    
    % Flocking parameters
    epsilon = params(1); a = params(2); b = params(3); c = params(4); d = params(5); h = params(6);

    e = abs(a - b) / sqrt(4*a*b) ;

    cAlpha = sigmaNormFun(c, epsilon) ;
    dAlpha = sigmaNormFun(d, epsilon) ;

    %%
    Pi = [xi;yi] ;
    Pj = [xj;yj] ;
    Pk = [xk;yk] ;
    Pl = [xl;yl] ;

    %%
    sigmaNormj = sigmaNormFun(Pj - Pi, epsilon) ;
    nij = gradSigmaFun(Pj - Pi, epsilon) ;
    
    sigmaNormk = sigmaNormFun(Pk - Pi, epsilon) ;
    nik = gradSigmaFun(Pk - Pi, epsilon) ;

    sigmaNorml = sigmaNormFun(Pl - Pi, epsilon) ;
    nil = gradSigmaFun(Pl - Pi, epsilon) ;

    %%
    sigma1j = sigma1Fun(sigmaNormj - dAlpha + e) ;
    sigma1k = sigma1Fun(sigmaNormk - dAlpha + e) ;
    sigma1l = sigma1Fun(sigmaNorml - dAlpha + e) ;
            
    %% Position
    phiAlphaj = 0.5 * bumpFcn(sigmaNormj/cAlpha,h) * ((a+b)*sigma1j + (a-b)) ;
    phiAlphanij = phiAlphaj.* nij ;
    
    phiAlphak = 0.5 * bumpFcn(sigmaNormk/cAlpha,h) * ((a+b)*sigma1k + (a-b)) ;
    phiAlphanik = phiAlphak.* nik ;

    phiAlphal = 0.5 * bumpFcn(sigmaNorml/cAlpha,h) * ((a+b)*sigma1l + (a-b)) ;
    phiAlphanil = phiAlphal.* nil ;

    phiAlpha = phiAlphanij + phiAlphanik + phiAlphanil;

    
end

== matlab function test_pi_av_flocking_xy_gazebo_2023a/Translational Control3/Flocking1/MATLAB Function1 ==
  data: eta input; phiAlpha input; phiAlpha_int input; ui_gamma input; yaw input; Ui_pos output size=3; ui_yaw output; KP input; eyaw output size=1; eyaw1 input; eyaw2 input; eyaw4 input

function [Ui_pos, ui_yaw, eyaw]  = ctrlLaw(eta, phiAlpha, phiAlpha_int, ui_gamma, yaw, KP, eyaw1, eyaw2, eyaw4)  %, phiBetak, bikobs, phiBetanei, bikve
    
    % Control gains and parameters
    Kx = KP(1); Ky = KP(2); Kz = KP(3);
    Kix = KP(4); Kiy = KP(5); Kiz = KP(6);
    Kyaw = KP(7); Kdyaw = KP(8);
    off = KP(9);

    eyaw = 0 - yaw(1);
    deyaw = 0 - yaw(2);


    ui_yaw = Kyaw*eyaw + Kdyaw*deyaw;
    hz_dot = ui_gamma(3,1) - eta(3,1);  %+ cBetaz * (phiBetak(3,1) + phiBetanei(3,1)) + cdBetaz * (bikobs(3,1) + bikve(3,1));

    if eyaw < off && eyaw > -off % && eyaw1 < off && eyaw1 > -off && eyaw2 < off && eyaw2 > -off && eyaw4 < off && eyaw4 > -off
        hx_dot = Kx * phiAlpha(1,1) + Kix * phiAlpha_int(1,1) + ui_gamma(1,1) - eta(1,1);  %+ cBetax * (phiBetak(1,1) + phiBetanei(1,1)) + cdBetax * (bikobs(1,1) + bikve(1,1));
        hy_dot = Ky * phiAlpha(2,1) + Kiy * phiAlpha_int(2,1) + ui_gamma(2,1) - eta(2,1);  %+ cBetay * (phiBetak(2,1) + phiBetanei(2,1)) + cdBetay * (bikobs(2,1) + bikve(2,1));
    else
        hx_dot = 0;
        hy_dot = 0;
    end
    

    Ui_pos = [hx_dot; hy_dot; hz_dot] ;
    

end

== matlab function test_pi_av_flocking_xy_gazebo_2023a/Translational Control3/Flocking1/MATLAB Function2 ==
  data: xi input; yi input; zi input; ui_gamma output; xr input; yr input; zr input; xr2 input; yr2 input; zr2 input; fig input; iep input size=3; ep output size=3; K_cts input
function [ui_gamma, ep] = naviFeedback(xi, yi, zi, xr, yr, zr, xr2, yr2, zr2, fig, iep, K_cts)
    
    Kpxy = K_cts(1); Kixy = K_cts(2);
    xminxy = K_cts(3); xmaxxy = K_cts(4);
    Kpz = K_cts(5); Kiz = K_cts(6);
    xminz = K_cts(7); xmaxz = K_cts(8);
    
    if fig == 1
        e_x = (xr - xi - 0.5) + (xr2 - xi - 1);
        e_y = (yr - yi - 0.5) + (yr2 - yi);
        e_z = (zr - zi + 0.1) + (zr2 - zi);
    elseif fig == 2
        e_x = (xr - xi + 0.5) + (xr2 - xi);
        e_y = (yr - yi - 0.5) + (yr2 - yi - 1);
        e_z = (zr - zi - 0.1) + (zr2 - zi);
    else
        e_x = (xr - xi + 0.5) + (xr2 - xi);
        e_y = (yr - yi - 0.5) + (yr2 - yi - 1);
        e_z = (zr - zi - 0.5) + (zr2 - zi - 0.6);
    end

    e_xy = [e_x;e_y];
    ep = [e_xy;e_z];
    
    ui_xy = satFcn_xy(Kpxy.*(e_xy), xminxy, xmaxxy) + satFcn_xy(Kixy.*([iep(1);iep(2)]), xminxy, xmaxxy) ;
    ui_z = satFcn_z(Kpz*(e_z), xminz, xmaxz) + satFcn_z(Kiz*(iep(3)), xminz, xmaxz) ;

    ui_gamma = [ui_xy;ui_z];    
    
end
